simulink model "Open_And_Closed_System"  (R2021a)
settings: Solver=VariableStepAuto  StartTime=0.0  StopTime=10.0  RelTol=1e-3
libraries: simulink x1
settings Model: Creator=lenovo  LastModifiedBy=lenovo

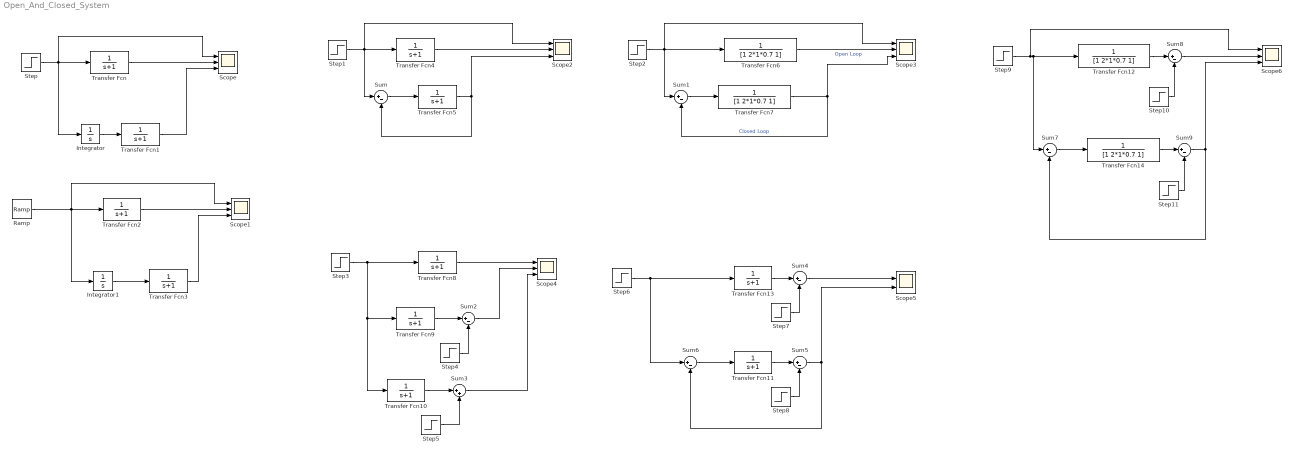
== system Open_And_Closed_System ==
  Integrator : Integrator
  Integrator1 : Integrator
  Ramp : simulink/Sources/Ramp  slope=1  start=0  InitialOutput=0
  Scope{,1..4,6} (6 alike) : Scope  NumInputPorts=3
  Scope5 : Scope  NumInputPorts=2
  Step{,1..3,6,9} (6 alike) : Step  SampleTime=0
  Step10 : Step  Time=3  After=-0.7  SampleTime=0
  Step11 : Step  Time=3  After=-.7  SampleTime=0
  Step{4..5,7..8} (4 alike) : Step  Time=3  After=0.7  SampleTime=0
  Sum{,1..2,4..9} (9 alike) : Sum  Inputs=|+-
  Sum3 : Sum  Inputs=|++
  Transfer Fcn{,1..5,8..11,13} (11 alike) : TransferFcn  Denominator=[1 1]
  Transfer Fcn{6..7,12,14} (4 alike) : TransferFcn  Denominator=[1 2*1*0.7 1]
  wires:
  Step/1 -> Scope/1, Integrator/1, Transfer Fcn/1
  Transfer Fcn/1 -> Scope/2
  Integrator/1 -> Transfer Fcn1/1
  Transfer Fcn1/1 -> Scope/3
  Transfer Fcn3/1 -> Scope1/3
  Integrator1/1 -> Transfer Fcn3/1
  Transfer Fcn2/1 -> Scope1/2
  Ramp/1 -> Transfer Fcn2/1, Integrator1/1, Scope1/1
  Transfer Fcn4/1 -> Scope2/2
  Step1/1 -> Scope2/1, Sum/1, Transfer Fcn4/1
  Sum/1 -> Transfer Fcn5/1
  Transfer Fcn5/1 -> Scope2/3, Sum/2
  Transfer Fcn7/1 -> Sum1/2, Scope3/3  "Closed Loop"
  Sum1/1 -> Transfer Fcn7/1
  Step2/1 -> Transfer Fcn6/1, Sum1/1, Scope3/1
  Transfer Fcn6/1 -> Scope3/2  "Open Loop"
  Transfer Fcn8/1 -> Scope4/1
  Sum2/1 -> Scope4/2
  Transfer Fcn9/1 -> Sum2/1
  Step4/1 -> Sum2/2
  Step5/1 -> Sum3/2
  Transfer Fcn10/1 -> Sum3/1
  Sum3/1 -> Scope4/3
  Step3/1 -> Transfer Fcn8/1, Transfer Fcn10/1, Transfer Fcn9/1
  Step6/1 -> Sum6/1, Transfer Fcn13/1
  Step7/1 -> Sum4/2
  Transfer Fcn13/1 -> Sum4/1
  Sum4/1 -> Scope5/1
  Sum5/1 -> Scope5/2, Sum6/2
  Transfer Fcn11/1 -> Sum5/1
  Step8/1 -> Sum5/2
  Sum6/1 -> Transfer Fcn11/1
  Step9/1 -> Sum7/1, Transfer Fcn12/1, Scope6/1
  Sum7/1 -> Transfer Fcn14/1
  Transfer Fcn12/1 -> Sum8/1
  Sum8/1 -> Scope6/2
  Step10/1 -> Sum8/2
  Step11/1 -> Sum9/2
  Transfer Fcn14/1 -> Sum9/1
  Sum9/1 -> Scope6/3, Sum7/2
